simulink model "SecRwRtStLgrstInwdOtwdCtrl"  (R2018b)
settings: Solver=FixedStepDiscrete  StartTime=0.0  StopTime=10.0  FixedStep=0.01  RelTol=1e-3
undefined symbols (not defined in the file or in its folder): KeSMSuMdMotFinshdTm_Val, KeSMSuMdRetryTm1_Val, KeSMSuModeReqDurgTm_Val
libraries: StCtrlLibBkRecln x1
settings Model: Creator=sn2xws  LastModifiedBy=sn55gm
settings Model: ModifiedHistory=|
  | 2024.10.14 V3.0.0 bitmask更换变量接口
  | 25.7.7 V3.13.0 Md61 Md62新增Retry口
  | 25.12.04 V3.14.0 Md12 防夹后退出
settings DataIOCC: SaveFormat=StructureWithTime
settings OptimizationCC: DefaultParameterBehavior=Inlined  EnhancedBackFolding=on  PassReuseOutputArgsAs=Individual arguments  ZeroExternalMemoryAtStartup=off  ZeroInternalMemoryAtStartup=off  OptimizeBlockOrder=speed  DifferentSizesBufferReuse=on  OptimizationCustomize=off
settings DebuggingCC: ParameterTunabilityLossMsg=error
settings ModelReferenceCC: ModelReferenceNumInstancesAllowed=Single
settings SFSimCC: MATLABDynamicMemAlloc=off
settings RTWCC: SystemTargetFile=autosar.tlc  GenCodeOnly=on  TemplateMakefile=ert_default_tmf  Description=AUTOSAR  GenerateReport=on  IncludeHyperlinkInReport=on  LaunchReport=on  GenerateTraceInfo=on  GenerateTraceReport=on  GenerateTraceReportSl=on  GenerateTraceReportSf=on  GenerateTraceReportEml=on
settings CodeAppCC: ForceParamTrailComments=on  IgnoreCustomStorageClasses=off  OperatorAnnotations=on  SimulinkDataObjDesc=on  SFDataObjDesc=on  InsertBlockDesc=on
settings STFCustomTargetCC: TargetLangStandard=C99 (ISO)  MultiwordLength=256  ParMdlRefBuildCompliant=on  CompOptLevelCompliant=on  IncludeMdlTerminateFcn=off  CombineOutputUpdateFcns=on  SuppressErrorStatus=on  ERTCustomFileBanners=on  SupportNonFinite=off  SupportComplex=off  SupportContinuousTime=off  SupportNonInlinedSFcns=off  RemoveResetFunc=on  MATLABClassNameForMDSCustomization=Simulink.SoftwareTarget.ERTCustomization  AutosarCompliant=on  UseToolchainInfoCompliant=on  LookupTableObjectStructAxisOrder=2,1,3,4,...  LUTObjectStructOrderEvenSpacing=Size,Table,Breakpoints  SystemTargetFile=autosar.tlc
settings ERTTargetCC: TargetLangStandard=C99 (ISO)  ConcurrentExecutionCompliant=off  IncludeMdlTerminateFcn=off  SuppressErrorStatus=on  SupportNonFinite=off  SupportComplex=off  ModelStepFunctionPrototypeControlCompliant=off  CPPClassGenCompliant=off  AutosarCompliant=on  LookupTableObjectStructAxisOrder=2,1,3,4,...  LUTObjectStructOrderEvenSpacing=Size,Table,Breakpoints  InlinedParameterPlacement=NonHierarchical  ERTCustomFileTemplate=example_file_process.tlc  ERTFilePackagingFormat=Compact

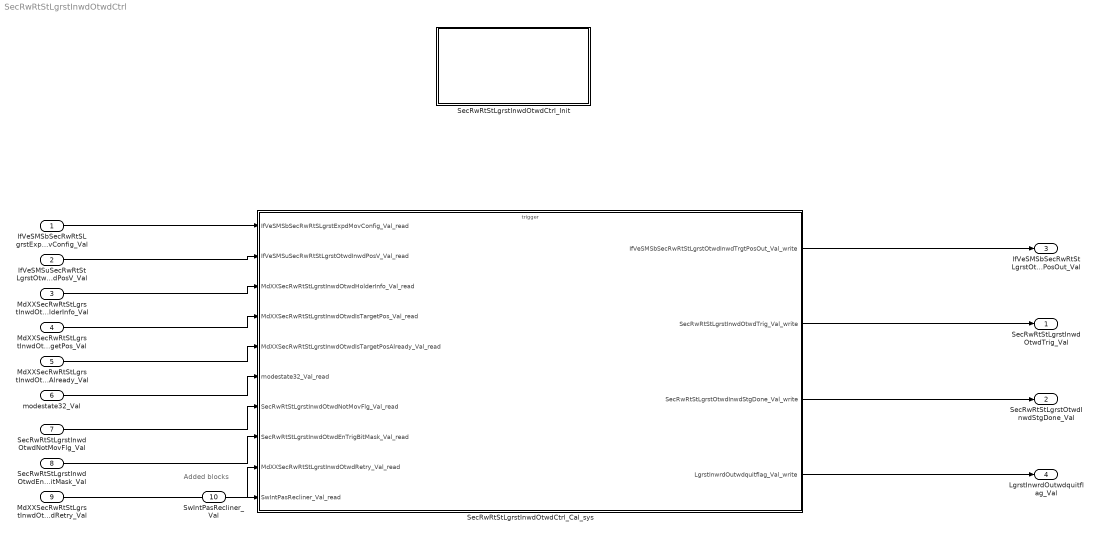
== system SecRwRtStLgrstInwdOtwdCtrl ==
  note: Added blocks
  IfVeSMSbSecRwRtSLgrstExpdMovConfig_Val : Inport  OutDataTypeStr=boolean  PortDimensions=1
  IfVeSMSuSecRwRtStLgrstOtwdInwdPosV_Val : Inport  Port=2  OutDataTypeStr=boolean  PortDimensions=1
  MdXXSecRwRtStLgrstInwdOtwdHolderInfo_Val : Inport  Port=3  OutDataTypeStr=uint32  PortDimensions=1
  MdXXSecRwRtStLgrstInwdOtwdIsTargetPos_Val : Inport  Port=4  OutDataTypeStr=uint32  PortDimensions=1
  MdXXSecRwRtStLgrstInwdOtwdIsTargetPosAlready_Val : Inport  Port=5  OutDataTypeStr=uint32  PortDimensions=1
  modestate32_Val : Inport  Port=6  OutDataTypeStr=uint32  PortDimensions=1
  SecRwRtStLgrstInwdOtwdNotMovFlg_Val : Inport  Port=7  OutDataTypeStr=boolean  PortDimensions=1
  SecRwRtStLgrstInwdOtwdEnTrigBitMask_Val : Inport  Port=8  OutDataTypeStr=uint32  PortDimensions=1
  MdXXSecRwRtStLgrstInwdOtwdRetry_Val : Inport  Port=9  OutDataTypeStr=uint32  PortDimensions=1
  SwIntPasRecliner_Val : Inport  Port=10  OutDataTypeStr=boolean  PortDimensions=1
  SecRwRtStLgrstInwdOtwdCtrl_Cal_sys : Subsystem
  SecRwRtStLgrstInwdOtwdCtrl_Init : Subsystem
  SecRwRtStLgrstInwdOtwdTrig_Val : Outport  OutDataTypeStr=boolean  PortDimensions=1
  SecRwRtStLgrstOtwdInwdStgDone_Val : Outport  Port=2  OutDataTypeStr=boolean  PortDimensions=1
  IfVeSMSbSecRwRtStLgrstOtwdInwdTrgtPosOut_Val : Outport  Port=3  OutDataTypeStr=boolean  PortDimensions=1
  LgrstInwrdOutwdquitflag_Val : Outport  Port=4  OutDataTypeStr=boolean  PortDimensions=1
  wires:
  IfVeSMSbSecRwRtSLgrstExpdMovConfig_Val/1 -> SecRwRtStLgrstInwdOtwdCtrl_Cal_sys/1(IfVeSMSbSecRwRtSLgrstExpdMovConfig_Val_read)
  IfVeSMSuSecRwRtStLgrstOtwdInwdPosV_Val/1 -> SecRwRtStLgrstInwdOtwdCtrl_Cal_sys/2(IfVeSMSuSecRwRtStLgrstOtwdInwdPosV_Val_read)
  MdXXSecRwRtStLgrstInwdOtwdHolderInfo_Val/1 -> SecRwRtStLgrstInwdOtwdCtrl_Cal_sys/3(MdXXSecRwRtStLgrstInwdOtwdHolderInfo_Val_read)
  MdXXSecRwRtStLgrstInwdOtwdIsTargetPos_Val/1 -> SecRwRtStLgrstInwdOtwdCtrl_Cal_sys/4(MdXXSecRwRtStLgrstInwdOtwdIsTargetPos_Val_read)
  MdXXSecRwRtStLgrstInwdOtwdIsTargetPosAlready_Val/1 -> SecRwRtStLgrstInwdOtwdCtrl_Cal_sys/5(MdXXSecRwRtStLgrstInwdOtwdIsTargetPosAlready_Val_read)
  modestate32_Val/1 -> SecRwRtStLgrstInwdOtwdCtrl_Cal_sys/6(modestate32_Val_read)
  SecRwRtStLgrstInwdOtwdNotMovFlg_Val/1 -> SecRwRtStLgrstInwdOtwdCtrl_Cal_sys/7(SecRwRtStLgrstInwdOtwdNotMovFlg_Val_read)
  SecRwRtStLgrstInwdOtwdCtrl_Cal_sys/1(IfVeSMSbSecRwRtStLgrstOtwdInwdTrgtPosOut_Val_write) -> IfVeSMSbSecRwRtStLgrstOtwdInwdTrgtPosOut_Val/1
  SecRwRtStLgrstInwdOtwdCtrl_Cal_sys/2(SecRwRtStLgrstInwdOtwdTrig_Val_write) -> SecRwRtStLgrstInwdOtwdTrig_Val/1
  SecRwRtStLgrstInwdOtwdCtrl_Cal_sys/3(SecRwRtStLgrstOtwdInwdStgDone_Val_write) -> SecRwRtStLgrstOtwdInwdStgDone_Val/1
  SecRwRtStLgrstInwdOtwdEnTrigBitMask_Val/1 -> SecRwRtStLgrstInwdOtwdCtrl_Cal_sys/8(SecRwRtStLgrstInwdOtwdEnTrigBitMask_Val_read)
  MdXXSecRwRtStLgrstInwdOtwdRetry_Val/1 -> SecRwRtStLgrstInwdOtwdCtrl_Cal_sys/9(MdXXSecRwRtStLgrstInwdOtwdRetry_Val_read)
  SecRwRtStLgrstInwdOtwdCtrl_Cal_sys/4(LgrstInwrdOutwdquitflag_Val_write) -> LgrstInwrdOutwdquitflag_Val/1
  SwIntPasRecliner_Val/1 -> SecRwRtStLgrstInwdOtwdCtrl_Cal_sys/10(SwIntPasRecliner_Val_read)

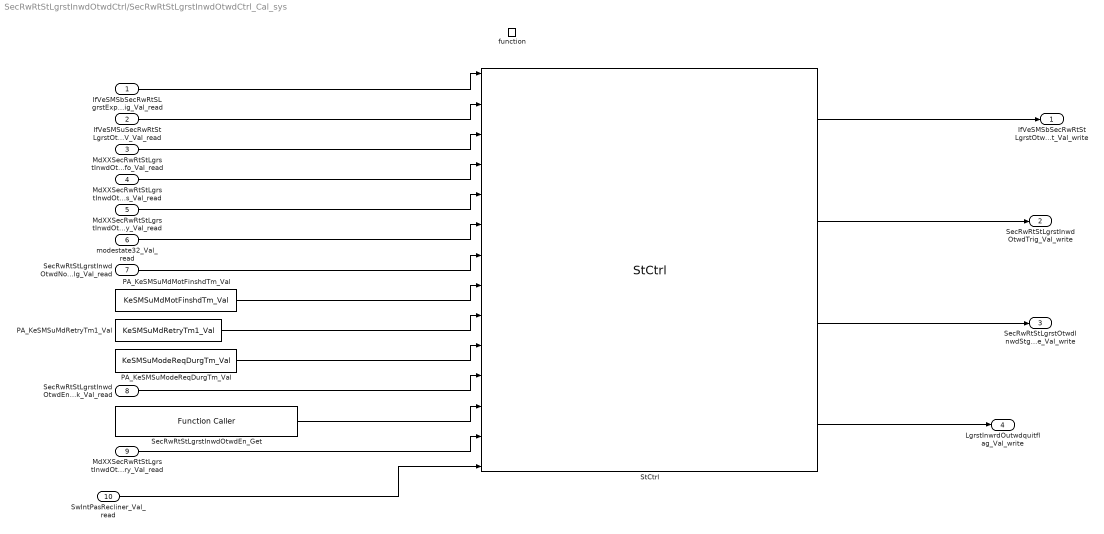
== system SecRwRtStLgrstInwdOtwdCtrl/SecRwRtStLgrstInwdOtwdCtrl_Cal_sys ==
  IfVeSMSbSecRwRtSLgrstExpdMovConfig_Val_read : Inport
  IfVeSMSuSecRwRtStLgrstOtwdInwdPosV_Val_read : Inport  Port=2
  MdXXSecRwRtStLgrstInwdOtwdHolderInfo_Val_read : Inport  Port=3
  MdXXSecRwRtStLgrstInwdOtwdIsTargetPos_Val_read : Inport  Port=4
  MdXXSecRwRtStLgrstInwdOtwdIsTargetPosAlready_Val_read : Inport  Port=5
  modestate32_Val_read : Inport  Port=6
  SecRwRtStLgrstInwdOtwdNotMovFlg_Val_read : Inport  Port=7
  SecRwRtStLgrstInwdOtwdEnTrigBitMask_Val_read : Inport  Port=8
  MdXXSecRwRtStLgrstInwdOtwdRetry_Val_read : Inport  Port=9
  SwIntPasRecliner_Val_read : Inport  Port=10
  function : TriggerPort  TriggerType=function-call  IsSimulinkFunction=on  FunctionName=SecRwRtStLgrstInwdOtwdCtrl_Cal  VariantControl=(inherit)
  PA_KeSMSuMdMotFinshdTm_Val : Constant  Value=KeSMSuMdMotFinshdTm_Val
  PA_KeSMSuMdRetryTm1_Val : Constant  Value=KeSMSuMdRetryTm1_Val
  PA_KeSMSuModeReqDurgTm_Val : Constant  Value=KeSMSuModeReqDurgTm_Val
  SecRwRtStLgrstInwdOtwdEn_Get : FunctionCaller  FunctionPrototype=data = SecRwRtStLgrstInwdOtwdEn_Get()  OutputArgumentSpecifications=uint32(1)
  StCtrl : StCtrlLibBkRecln/StCtrl  SystemSampleTime=-1
  IfVeSMSbSecRwRtStLgrstOtwdInwdTrgtPosOut_Val_write : Outport
      settings: EnsureOutportIsVirtual=on
  SecRwRtStLgrstInwdOtwdTrig_Val_write : Outport  Port=2
      settings: EnsureOutportIsVirtual=on
  SecRwRtStLgrstOtwdInwdStgDone_Val_write : Outport  Port=3
      settings: EnsureOutportIsVirtual=on
  LgrstInwrdOutwdquitflag_Val_write : Outport  Port=4
      settings: EnsureOutportIsVirtual=on
  wires:
  StCtrl/1 -> IfVeSMSbSecRwRtStLgrstOtwdInwdTrgtPosOut_Val_write/1
  StCtrl/2 -> SecRwRtStLgrstInwdOtwdTrig_Val_write/1
  StCtrl/3 -> SecRwRtStLgrstOtwdInwdStgDone_Val_write/1
  SecRwRtStLgrstInwdOtwdEnTrigBitMask_Val_read/1 -> StCtrl/11
  SecRwRtStLgrstInwdOtwdEn_Get/1 -> StCtrl/12
  PA_KeSMSuModeReqDurgTm_Val/1 -> StCtrl/10
  PA_KeSMSuMdMotFinshdTm_Val/1 -> StCtrl/8
  PA_KeSMSuMdRetryTm1_Val/1 -> StCtrl/9
  modestate32_Val_read/1 -> StCtrl/6
  SecRwRtStLgrstInwdOtwdNotMovFlg_Val_read/1 -> StCtrl/7
  MdXXSecRwRtStLgrstInwdOtwdIsTargetPos_Val_read/1 -> StCtrl/4
  MdXXSecRwRtStLgrstInwdOtwdIsTargetPosAlready_Val_read/1 -> StCtrl/5
  IfVeSMSbSecRwRtSLgrstExpdMovConfig_Val_read/1 -> StCtrl/1
  IfVeSMSuSecRwRtStLgrstOtwdInwdPosV_Val_read/1 -> StCtrl/2
  MdXXSecRwRtStLgrstInwdOtwdHolderInfo_Val_read/1 -> StCtrl/3
  MdXXSecRwRtStLgrstInwdOtwdRetry_Val_read/1 -> StCtrl/13
  StCtrl/4 -> LgrstInwrdOutwdquitflag_Val_write/1
  SwIntPasRecliner_Val_read/1 -> StCtrl/14

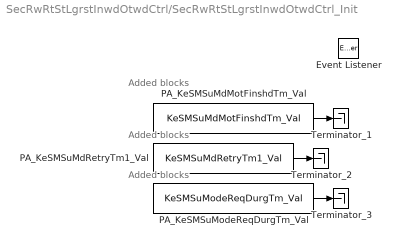
== system SecRwRtStLgrstInwdOtwdCtrl/SecRwRtStLgrstInwdOtwdCtrl_Init ==
  note: Added blocks
  note: Added blocks
  note: Added blocks
  Event Listener : EventListener  EventName=reset
  PA_KeSMSuMdMotFinshdTm_Val : Constant  Value=KeSMSuMdMotFinshdTm_Val
  PA_KeSMSuMdRetryTm1_Val : Constant  Value=KeSMSuMdRetryTm1_Val
  PA_KeSMSuModeReqDurgTm_Val : Constant  Value=KeSMSuModeReqDurgTm_Val
  Terminator_1 : Terminator
  Terminator_2 : Terminator
  Terminator_3 : Terminator
  wires:
  PA_KeSMSuMdMotFinshdTm_Val/1 -> Terminator_1/1
  PA_KeSMSuMdRetryTm1_Val/1 -> Terminator_2/1
  PA_KeSMSuModeReqDurgTm_Val/1 -> Terminator_3/1
